simulink model "cic"  (Simulink 7.2)
settings: Solver=FixedStepDiscrete  StartTime=0.0  StopTime=100  RelTol=1e-3
undefined symbols (not defined in the file or in its folder): dfilt, get
libraries: dspsrcs4 x4, dspmathops x4, dsparch4 x4, simulink_extras x1, dspsnks4 x1
settings Model: Creator=Administrator  LastModifiedBy=Administrator
settings DebuggingCC: SigSpecEnsureSampleTimeMsg=none  StrictBusMsg=ErrorLevel1

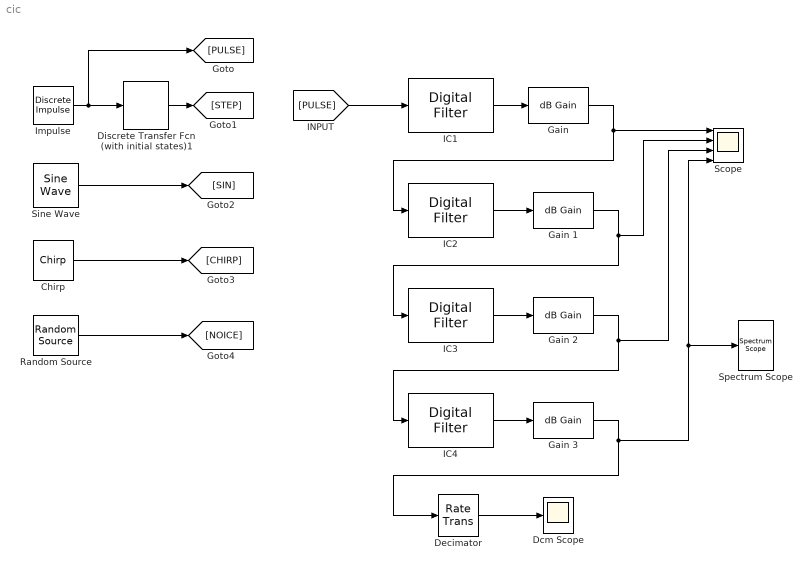
== system cic ==
  Chirp : dspsrcs4/Chirp  sweep=Linear  mode=Unidirectional  f0=0  f1=0.5  t1=10000  Tsweep=10000  phase=0  Ts=1  spf=1  datatype=Double
  Dcm Scope : Scope
      settings: TickLabels=on  TimeRange=20.6726825266612  YMin=-2  YMax=2  Decimation=2  SampleInput=on  SampleTime=6
  Decimator : RateTransition  Integrity=off  OutPortSampleTime=6
  Discrete Transfer Fcn (with initial states)1 : simulink_extras/Additional Discrete/Discrete Transfer Fcn (with initial states)  SystemSampleTime=-1  N=[1]  D=[1 -1]  X0=[ ]  TS=1
  Gain {,1..3} (4 alike) : dspmathops/dB Gain  SystemSampleTime=-1  dB=-21.58  intype=Amplitude
  IC1 : dsparch4/Digital Filter  DialogController=dspdialog.DigitalFilter  DialogControllerArgs=DataTag1  TypePopup=IIR (poles & zeros)  IIRFiltStruct=Direct form I  AllPoleFiltStruct=Direct form  FIRFiltStruct=Direct form  CoeffSource=Specify via dialog  NumCoeffs=[1 0 0 0 0 0 0 0 0 0 0 0 -1]  DenCoeffs=[1 -1]  BiQuadCoeffs=[1 0.3 0.4 1 0.1 0.2]  LatticeCoeffs=[0.2 0.4]  denIgnore=on  FiltPerSampPopup=One filter per frame  IC=0  ICnum=0  ICden=0  roundingMode=Floor  overflowMode=off  ScaleValues=1  scaleValueFracLength=14  stageInFracLength=15  stageOutFracLength=15  FilterSource=Specify via dialog  dfiltObjectName=dfilt.dffir([1 2 1])
  IC2 : dsparch4/Digital Filter  DialogController=dspdialog.DigitalFilter  DialogControllerArgs=DataTag3  TypePopup=IIR (poles & zeros)  IIRFiltStruct=Direct form I  AllPoleFiltStruct=Direct form  FIRFiltStruct=Direct form  CoeffSource=Specify via dialog  NumCoeffs=[1 0 0 0 0 0 0 0 0 0 0 0 -1]  DenCoeffs=[1 -1]  BiQuadCoeffs=[1 0.3 0.4 1 0.1 0.2]  LatticeCoeffs=[0.2 0.4]  denIgnore=on  FiltPerSampPopup=One filter per frame  IC=0  ICnum=0  ICden=0  roundingMode=Floor  overflowMode=off  ScaleValues=1  scaleValueFracLength=14  stageInFracLength=15  stageOutFracLength=15  FilterSource=Specify via dialog  dfiltObjectName=dfilt.dffir([1 2 1])
  IC3 : dsparch4/Digital Filter  DialogController=dspdialog.DigitalFilter  DialogControllerArgs=DataTag5  TypePopup=IIR (poles & zeros)  IIRFiltStruct=Direct form I  AllPoleFiltStruct=Direct form  FIRFiltStruct=Direct form  CoeffSource=Specify via dialog  NumCoeffs=[1 0 0 0 0 0 0 0 0 0 0 0 -1]  DenCoeffs=[1 -1]  BiQuadCoeffs=[1 0.3 0.4 1 0.1 0.2]  LatticeCoeffs=[0.2 0.4]  denIgnore=on  FiltPerSampPopup=One filter per frame  IC=0  ICnum=0  ICden=0  roundingMode=Floor  overflowMode=off  ScaleValues=1  scaleValueFracLength=14  stageInFracLength=15  stageOutFracLength=15  FilterSource=Specify via dialog  dfiltObjectName=dfilt.dffir([1 2 1])
  IC4 : dsparch4/Digital Filter  DialogController=dspdialog.DigitalFilter  DialogControllerArgs=DataTag7  TypePopup=IIR (poles & zeros)  IIRFiltStruct=Direct form I  AllPoleFiltStruct=Direct form  FIRFiltStruct=Direct form  CoeffSource=Specify via dialog  NumCoeffs=[1 0 0 0 0 0 0 0 0 0 0 0 -1]  DenCoeffs=[1 -1]  BiQuadCoeffs=[1 0.3 0.4 1 0.1 0.2]  LatticeCoeffs=[0.2 0.4]  denIgnore=on  FiltPerSampPopup=One filter per frame  IC=0  ICnum=0  ICden=0  roundingMode=Floor  overflowMode=off  ScaleValues=1  scaleValueFracLength=14  stageInFracLength=15  stageOutFracLength=15  FilterSource=Specify via dialog  dfiltObjectName=dfilt.dffir([1 2 1])
  Impulse : dspsrcs4/Discrete  Impulse  Delay=1  SampleTime=1  FrameSample=1  dataType=double  isSigned=on  wordLen=16  udDataType=sfix(16)  fracBitsMode=Best precision  numFracBits=15
  Random Source : dspsrcs4/Random Source  SrcType=Gaussian  NormMethod=Ziggurat  CltLength=12  MinVal=0  MaxVal=1  MeanVal=0  VarVal=1  RepMode=Specify seed  rawSeed=1234567  IsInherit=off  SampMode=Discrete  SampTime=1  SampFrame=1  DataType=Double  OutComplex=Real
  Scope : Scope  NumInputPorts=4
      settings: TimeRange=50000  YMin=-3~-5~-5~-5  YMax=3~5~5~5  SampleInput=on  SampleTime=1
  Sine Wave : dspsrcs4/Sine Wave  Amplitude=1  Frequency=0/6 + 1.01/24  Phase=0  SampleMode=Discrete  OutComplex=Real  CompMethod=Trigonometric fcn  TableSize=Speed  SampleTime=1  SamplesPerFrame=1  dataType=double  wordLen=16  udDataType=sfix(16)  fracBitsMode=Best precision  numFracBits=15  ResetState=Restart at time zero
  Spectrum Scope : dspsnks4/Spectrum Scope  DialogController=dspdialog.SpectrumScope  DialogControllerArgs=DataTag9  SystemSampleTime=-1  ScopeProperties=on  Domain=Frequency  HorizSpan=1  UseBuffer=on  BufferSize=1024  Overlap=0  inpFftLenInherit=on  FFTlength=1024  numAvg=100  DisplayProperties=off  AxisGrid=on  Memory=off  FrameNumber=on  AxisLegend=off  AxisZoom=off  OpenScopeAtSimStart=off  OpenScopeImmediately=off  FigPos=get(0,'defaultfigureposition')  AxisProperties=off  XUnits=Hertz  XRange=[0...Fs/2]  XDisplay=0  InheritXIncr=on  XIncr=1.0  XLabel=Samples  XLimit=Auto  YUnits=dB  XMax=1  XMin=0  YLabel=Magnitude-squared, dB  LineProperties=off  wintypeSpecScope=Hann  RsSpecScope=50  betaSpecScope=5  winsampSpecScope=Periodic
      settings: YMin=-100  YMax=10
  wires:
  Impulse/1 -> Discrete Transfer Fcn (with initial states)1/1, [PULSE]
  Discrete Transfer Fcn (with initial states)1/1 -> [STEP]
  Sine Wave/1 -> [SIN]
  Random Source/1 -> [NOICE]
  Chirp/1 -> [CHIRP]
  [PULSE] -> IC1/1
  IC1/1 -> "Gain "/1
  "Gain "/1 -> IC2/1, Scope/1
  IC2/1 -> Gain 1/1
  IC3/1 -> Gain 2/1
  Gain 2/1 -> IC4/1, Scope/3
  Gain 1/1 -> IC3/1, Scope/2
  IC4/1 -> Gain 3/1
  Gain 3/1 -> Decimator/1, Scope/4, Spectrum Scope/1
  Decimator/1 -> Dcm Scope/1
